simulink model "s_tanks_3"  (Simulink 7.7)
settings: Solver=ode4  StartTime=0.0  StopTime=60  FixedStep=0.002  RelTol=1e-3
values from neighbouring files (symbols this model uses):
  gamma = Ai2 / ( Ai1 + Ai2 )    [d_tanks_3.m]
  Kff_2 = Ao2^2*(1-gamma)^2/Ao1^2    [d_tanks_3.m]
  Ki_2 = K(3)    [d_tanks_3.m]
  Kp_1 = K(1)    [d_tanks_3.m]
  Kp_2 = K(2)    [d_tanks_3.m]
undefined symbols (not defined in the file or in its folder): Ao1, Ao2, At1, At2, g, Kp, L20, LR_1_MAX, MAX_L2_WDUP, TS, VMAX_AMP
settings Model: Creator=MLevis  LastModifiedBy=pmartin  ExtModeTrigDuration=60000
settings SolverCC: PositivePriorityOrder=on
settings OptimizationCC: InitFltsAndDblsToZero=on
settings DebuggingCC: SaveWithParameterizedLinksMsg=none  StrictBusMsg=Warning
settings RTWCC: SystemTargetFile=quarc_windows.tlc  TemplateMakefile=quarc_default_tmf  Description=QuaRC Win32 Target  ProcessScript=quarc_windows_make_rtw_hook
settings STFCustomTargetCC: TargetFcnLib=ansi_tfl_tmw.mat  TargetPreCompLibLocation=C:\PROGRA~3\QUARC\lib\2012b\windows\release  GeneratePreprocessorConditionals=Disable all  SystemTargetFile=quarc_windows.tlc
settings GRTTargetCC: TargetFcnLib=ansi_tfl_tmw.mat  TargetPreCompLibLocation=C:\PROGRA~3\QUARC\lib\2012b\windows\release  ParMdlRefBuildCompliant=off  CompOptLevelCompliant=off  MatFileLogging=off  ExtMode=on  ExtModeMexFile=quarc_comm

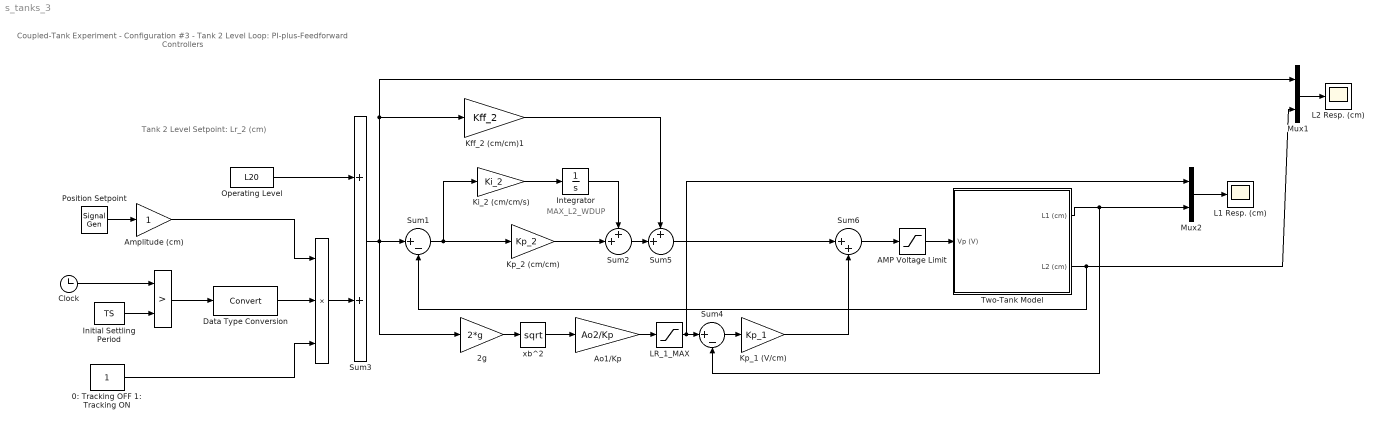
== system s_tanks_3 ==
  note: Coupled-Tank Experiment
      | - Configuration #3 -
      | Tank 2 Level Loop:
      | PI-plus-Feedforward Controllers
  note: Tank 2 Level Setpoint:
      | Lr_2 (cm)
  note: MAX_L2_WDUP
  "   " : Product  Inputs=3  SaturateOnIntegerOverflow=on  RndMeth=Zero  InputSameDT=on  OutDataTypeStr=Inherit: Same as first input
  "    " : RelationalOperator  Operator=>  InputSameDT=on
  0: Tracking OFF 1: Tracking ON : Constant
  2g : Gain  Gain=2*g  SaturateOnIntegerOverflow=on  OutDataTypeStr=Inherit: Same as input  ParamDataTypeStr=Inherit: Same as input
  AMP Voltage Limit : Saturate  UpperLimit=VMAX_AMP  LowerLimit=0
  Amplitude (cm) : Gain  SaturateOnIntegerOverflow=on  OutDataTypeStr=Inherit: Same as input  ParamDataTypeStr=Inherit: Same as input
  Ao1/Kp : Gain  Gain=Ao2/Kp  SaturateOnIntegerOverflow=on  OutDataTypeStr=Inherit: Same as input  ParamDataTypeStr=Inherit: Same as input
  Clock : Clock
  Data Type Conversion : DataTypeConversion
  Initial Settling Period : Constant  Value=TS
  Integrator : Integrator  LimitOutput=on  UpperSaturationLimit=MAX_L2_WDUP  LowerSaturationLimit=- MAX_L2_WDUP
  Kff_2 (cm/cm)1 : Gain  Gain=Kff_2  SaturateOnIntegerOverflow=on  OutDataTypeStr=Inherit: Same as input  ParamDataTypeStr=Inherit: Same as input
  Ki_2 (cm/cm/s) : Gain  Gain=Ki_2  SaturateOnIntegerOverflow=on  OutDataTypeStr=Inherit: Same as input  ParamDataTypeStr=Inherit: Same as input
  Kp_1 (V/cm) : Gain  Gain=Kp_1  SaturateOnIntegerOverflow=on  OutDataTypeStr=Inherit: Same as input  ParamDataTypeStr=Inherit: Same as input
  Kp_2 (cm/cm) : Gain  Gain=Kp_2  SaturateOnIntegerOverflow=on  OutDataTypeStr=Inherit: Same as input  ParamDataTypeStr=Inherit: Same as input
  L1 Resp. (cm) : Scope
      settings: TickLabels=on  TimeRange=60  YMin=0  YMax=30  SaveName=data_L1
  L2 Resp. (cm) : Scope
      settings: TickLabels=on  TimeRange=60  YMin=12  YMax=17  SaveName=data_L2
  LR_1_MAX : Saturate  UpperLimit=LR_1_MAX  LowerLimit=0
  Mux1 : Mux  Inputs=2
  Mux2 : Mux  Inputs=2
  Operating Level : Constant  Value=L20
  Position Setpoint : SignalGenerator  WaveForm=square  Frequency=0.018
  Sum1 : Sum  Inputs=|+-  SaturateOnIntegerOverflow=on  InputSameDT=on  OutDataTypeStr=Inherit: Same as first input
  Sum2 : Sum  Inputs=++|  SaturateOnIntegerOverflow=on  InputSameDT=on  OutDataTypeStr=Inherit: Same as first input
  Sum3 : Sum  SaturateOnIntegerOverflow=on  InputSameDT=on  OutDataTypeStr=Inherit: Same as first input
  Sum4 : Sum  Inputs=|+-  SaturateOnIntegerOverflow=on  InputSameDT=on  OutDataTypeStr=Inherit: Same as first input
  Sum5 : Sum  Inputs=++|  SaturateOnIntegerOverflow=on  InputSameDT=on  OutDataTypeStr=Inherit: Same as first input
  Sum6 : Sum  Inputs=|++  SaturateOnIntegerOverflow=on  InputSameDT=on  OutDataTypeStr=Inherit: Same as first input
  Two-Tank Model : Subsystem
  xb^2 : Math  Operator=sqrt  SaturateOnIntegerOverflow=on
  wires:
  Mux2/1 -> L1 Resp. (cm)/1
  Position Setpoint/1 -> Amplitude (cm)/1
  0: Tracking OFF 1: Tracking ON/1 -> "   "/3
  "   "/1 -> Sum3/2
  Operating Level/1 -> Sum3/1
  Sum1/1 -> Kp_2 (cm/cm)/1, Ki_2 (cm/cm/s)/1
  Ki_2 (cm/cm/s)/1 -> Integrator/1
  Kp_2 (cm/cm)/1 -> Sum2/2
  Integrator/1 -> Sum2/1
  Sum2/1 -> Sum5/2
  Kff_2 (cm/cm)1/1 -> Sum5/1
  Sum3/1 -> Sum1/1, 2g/1, Kff_2 (cm/cm)1/1, Mux1/1
  Mux1/1 -> L2 Resp. (cm)/1
  Initial Settling Period/1 -> "    "/2
  Clock/1 -> "    "/1
  Amplitude (cm)/1 -> "   "/1
  "    "/1 -> Data Type Conversion/1
  Data Type Conversion/1 -> "   "/2
  AMP Voltage Limit/1 -> Two-Tank Model/1(Vp (V))
  xb^2/1 -> Ao1/Kp/1
  2g/1 -> xb^2/1
  Two-Tank Model/2(L2 (cm)) -> Sum1/2, Mux1/2
  Ao1/Kp/1 -> LR_1_MAX/1
  Two-Tank Model/1(L1 (cm)) -> Sum4/2, Mux2/2
  Sum4/1 -> Kp_1 (V/cm)/1
  Sum5/1 -> Sum6/1
  Sum6/1 -> AMP Voltage Limit/1
  LR_1_MAX/1 -> Sum4/1, Mux2/1
  Kp_1 (V/cm)/1 -> Sum6/2

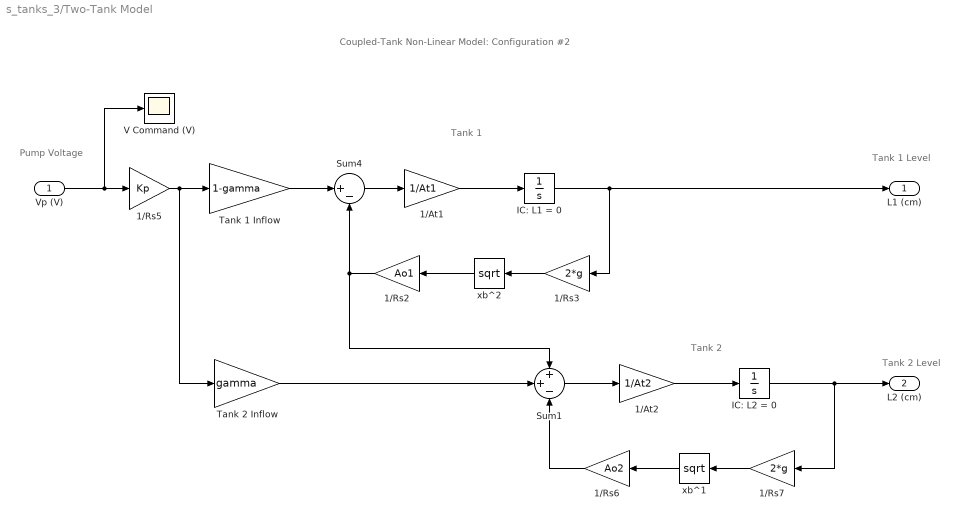
== system s_tanks_3/Two-Tank Model ==
  note: Pump
      | Voltage
  note: Tank 1 Level
  note: Tank 2 Level
  note: Tank 2
  note: Tank 1
  note: Coupled-Tank Non-Linear Model:
      | Configuration #2
  Vp (V) : Inport
  1/At1 : Gain  Gain=1/At1  SaturateOnIntegerOverflow=on  OutDataTypeStr=Inherit: Same as input  ParamDataTypeStr=Inherit: Same as input
  1/At2 : Gain  Gain=1/At2  SaturateOnIntegerOverflow=on  OutDataTypeStr=Inherit: Same as input  ParamDataTypeStr=Inherit: Same as input
  1/Rs2 : Gain  Gain=Ao1  SaturateOnIntegerOverflow=on  OutDataTypeStr=Inherit: Same as input  ParamDataTypeStr=Inherit: Same as input
  1/Rs3 : Gain  Gain=2*g  SaturateOnIntegerOverflow=on  OutDataTypeStr=Inherit: Same as input  ParamDataTypeStr=Inherit: Same as input
  1/Rs5 : Gain  Gain=Kp  SaturateOnIntegerOverflow=on  OutDataTypeStr=Inherit: Same as input  ParamDataTypeStr=Inherit: Same as input
  1/Rs6 : Gain  Gain=Ao2  SaturateOnIntegerOverflow=on  OutDataTypeStr=Inherit: Same as input  ParamDataTypeStr=Inherit: Same as input
  1/Rs7 : Gain  Gain=2*g  SaturateOnIntegerOverflow=on  OutDataTypeStr=Inherit: Same as input  ParamDataTypeStr=Inherit: Same as input
  IC: L1 = 0 : Integrator
  IC: L2 = 0 : Integrator
  Sum1 : Sum  Inputs=++-  SaturateOnIntegerOverflow=on  InputSameDT=on  OutDataTypeStr=Inherit: Same as first input
  Sum4 : Sum  Inputs=|+-  SaturateOnIntegerOverflow=on  InputSameDT=on  OutDataTypeStr=Inherit: Same as first input
  Tank 1 Inflow : Gain  Gain=1-gamma
  Tank 2 Inflow : Gain  Gain=gamma
  V Command (V) : Scope
      settings: TickLabels=on  TimeRange=1.000000  YMin=-1  YMax=1  SaveName=ScopeData2
  xb^1 : Math  Operator=sqrt  SaturateOnIntegerOverflow=on
  xb^2 : Math  Operator=sqrt  SaturateOnIntegerOverflow=on
  L1 (cm) : Outport  InitialOutput=0
  L2 (cm) : Outport  Port=2  InitialOutput=0
  wires:
  1/Rs7/1 -> xb^1/1
  xb^1/1 -> 1/Rs6/1
  IC: L2 = 0/1 -> L2 (cm)/1, 1/Rs7/1
  1/At2/1 -> IC: L2 = 0/1
  Sum1/1 -> 1/At2/1
  1/Rs3/1 -> xb^2/1
  xb^2/1 -> 1/Rs2/1
  1/Rs2/1 -> Sum4/2, Sum1/1
  IC: L1 = 0/1 -> L1 (cm)/1, 1/Rs3/1
  1/At1/1 -> IC: L1 = 0/1
  Sum4/1 -> 1/At1/1
  Vp (V)/1 -> 1/Rs5/1, V Command (V)/1
  1/Rs6/1 -> Sum1/3
  1/Rs5/1 -> Tank 1 Inflow/1, Tank 2 Inflow/1
  Tank 1 Inflow/1 -> Sum4/1
  Tank 2 Inflow/1 -> Sum1/2
